simulink model "rpend_dick"  (R2015b)
settings: Solver=FixedStepDiscrete  StartTime=0.0  StopTime=10  FixedStep=h  RelTol=1e-3
model workspace: external: MATLAB File par_struct.m (data not in the file)
values from neighbouring files (symbols this model uses):
  adingain = [adingain 1 1 1 1 1]    [hwinit.m]
  adinoffs = [adinoffs 0 0 0 0 0]    [hwinit.m]
  daoutgain = 1*[-6]    [hwinit.m]
  daoutoffs = [0.00]    [hwinit.m]
undefined symbols (not defined in the file or in its folder): discr_sys, h, K, L
settings Model: Creator=rbabuska  LastModifiedBy=dnieuwenhuizen
settings DataIOCC: SaveFormat=Array  SignalLoggingName=sigsOut
settings OptimizationCC: BooleanDataType=off  ExpressionDepthLimit=2147483647  InitFltsAndDblsToZero=on
settings DebuggingCC: SaveWithParameterizedLinksMsg=none  SignalResolutionControl=TryResolveAllWithWarning  MultiTaskDSMMsg=warning  MultiTaskCondExecSysMsg=none  StateNameClashWarn=warning
settings HardwareCC: ProdBitPerPointer=32  ProdLargestAtomicFloat=None  ProdIntDivRoundTo=Undefined  ProdEndianess=Unspecified  ProdWordSize=32  ProdHWDeviceType=32-bit Generic  TargetUnknown=on
settings GRTTargetCC: TargetFcnLib=ansi_tfl_tmw.mat  GeneratePreprocessorConditionals=Disable all  CombineOutputUpdateFcns=off  GRTInterface=on
settings ConfigComp: CovModelRefEnable=Off

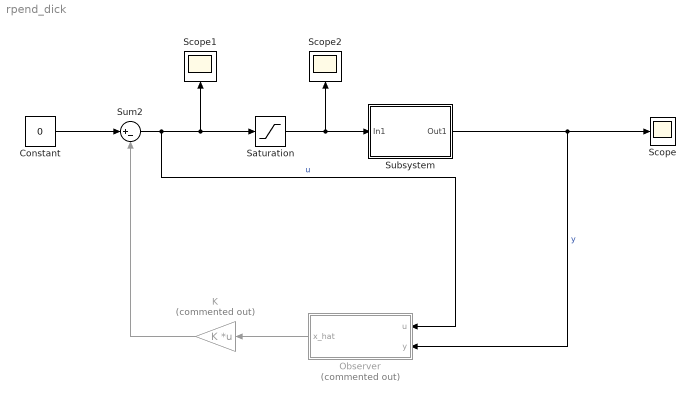
== system rpend_dick ==
  Constant : Constant  Value=0  SampleTime=h
  K : Gain  Commented=on  Gain=K  Multiplication=Matrix(K*u)
  Observer : Subsystem  Commented=on
  Saturation : Saturate  UpperLimit=0.00000001  LowerLimit=-0.0000001
  Scope : Scope
  Scope1 : Scope
  Scope2 : Scope
  Subsystem : Subsystem
      mask Display: disp('Rotational\nPendulum')
  Sum2 : Sum  Inputs=|+-
  wires:
  Saturation/1 -> Subsystem/1(In1), Scope2/1
  Subsystem/1(Out1) -> Observer/2(y), Scope/1  "y"
  Constant/1 -> Sum2/1
  K/1 -> Sum2/2
  Sum2/1 -> Observer/1(u), Saturation/1, Scope1/1  "u"
  Observer/1(x_hat) -> K/1

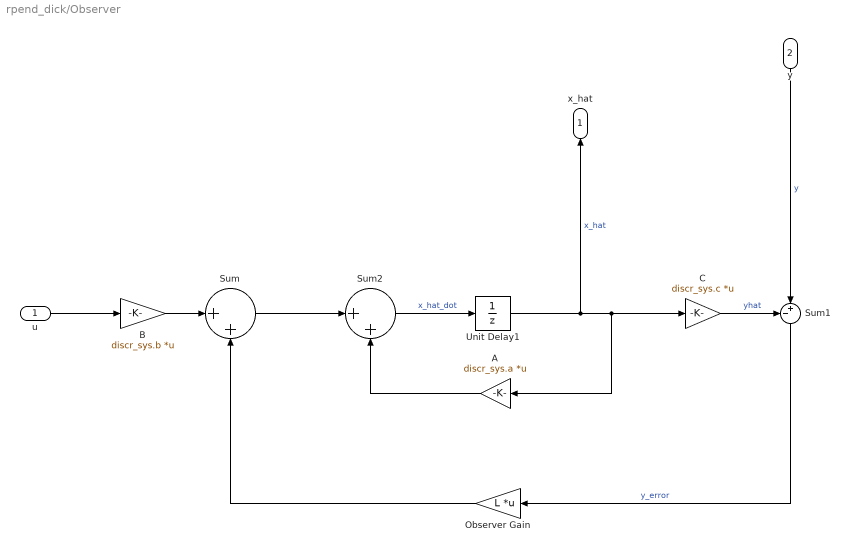
== system rpend_dick/Observer ==
  u : Inport
  y : Inport  Port=2
  A : Gain  Gain=discr_sys.a  Multiplication=Matrix(K*u)
  B : Gain  Gain=discr_sys.b  Multiplication=Matrix(K*u)
  C : Gain  Gain=discr_sys.c  Multiplication=Matrix(K*u)
  Observer Gain : Gain  Gain=L  Multiplication=Matrix(K*u)
  Sum : Sum  Inputs=|++
  Sum1 : Sum  Inputs=-+|
  Sum2 : Sum  Inputs=|++
  Unit Delay1 : UnitDelay  SampleTime=h
  x_hat : Outport
  wires:
  Observer Gain/1 -> Sum/2
  u/1 -> B/1
  B/1 -> Sum/1
  Sum/1 -> Sum2/1
  Sum2/1 -> Unit Delay1/1  "x_hat_dot"
  Unit Delay1/1 -> x_hat/1, C/1, A/1  "x_hat"
  A/1 -> Sum2/2
  C/1 -> Sum1/1  "yhat"
  Sum1/1 -> Observer Gain/1  "y_error"
  y/1 -> Sum1/2  "y"

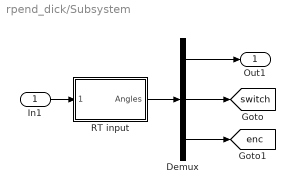
== system rpend_dick/Subsystem ==
  In1 : Inport
  Demux : Demux  Outputs=[2 4 1]
  RT input : Subsystem  mask{Ts=h, channels=[6 7]}
      mask prompts: Ts "Sample time [s]:"; channels "Channels to read (e.g., [6 7])"
      mask init:
      | hwinit;
      | 
      | % initialize FPGA
      | fugihandle = fugiboard('Open', 'Pendulum1');
      | fugihandle.WatchdogTimeout = 0.5;
      | fugiboard('SetParams', fugihandle);
      | fugiboard('Write', fugihandle, 0, 0, 0, 0);  % dummy write to sync interface board
      | fugiboard('Write', fugihandle, 5, 1, 0, 0);  % reset position, activate relay
      | data = fugiboard('Read', fugihandle);        % get version info from FPGA
      | % model = bitshift(data(1), -5); 
      | % version = bitand(data(1), 31);
      | % disp(sprintf('FPGA setup %d, version %d', model, version)); % for the B&P it should say 1 1, or else there is a problem
      | fugiboard('Write', fugihandle, 0, 1, 0, 0);  % end reset
      | pause(0.1);                         % give relay some time to respond
      mask Display: disp('Rotational\nPendulum')
  Out1 : Outport
  tag scope: enc=global, switch=global
  wires:
  RT input/1(Angles) -> Demux/1
  Demux/1 -> Out1/1
  Demux/2 -> [switch]
  Demux/3 -> [enc]
  In1/1 -> RT input/1(Motors)

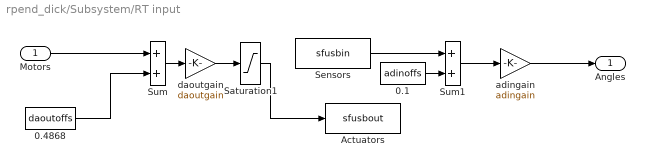
== system rpend_dick/Subsystem/RT input ==
  Motors : Inport
  0.1 : Constant  Value=adinoffs
  0.4868 : Constant  Value=daoutoffs
  Actuators : S-Function  FunctionName=sfusbout  Parameters=Ts, fugihandle  SFunctionDeploymentMode=off  EnableBusSupport=off
  Saturation1 : Saturate  UpperLimit=10  LowerLimit=-10
  Sensors : S-Function  FunctionName=sfusbin  Parameters=Ts, fugihandle, channels  SFunctionDeploymentMode=off  EnableBusSupport=off
  Sum : Sum  SaturateOnIntegerOverflow=on  InputSameDT=on  OutDataTypeStr=Inherit: Same as first input
  Sum1 : Sum  SaturateOnIntegerOverflow=on  InputSameDT=on  OutDataTypeStr=Inherit: Same as first input
  adingain : Gain  Gain=adingain  SaturateOnIntegerOverflow=on  OutDataTypeStr=Inherit: Same as input  ParamDataTypeStr=Inherit: Same as input
  daoutgain : Gain  Gain=daoutgain  SaturateOnIntegerOverflow=on  OutDataTypeStr=Inherit: Same as input  ParamDataTypeStr=Inherit: Same as input
  Angles : Outport
  wires:
  Sum/1 -> daoutgain/1
  0.4868/1 -> Sum/2
  Motors/1 -> Sum/1
  Sum1/1 -> adingain/1
  0.1/1 -> Sum1/2
  Sensors/1 -> Sum1/1
  adingain/1 -> Angles/1
  Saturation1/1 -> Actuators/1
  daoutgain/1 -> Saturation1/1
